simulink model "testemplanner_cs"  (R2020a)
settings: Solver=ode5  StartTime=0.0  StopTime=24  FixedStep=1/1000  RelTol=1e-3
PreLoadFcn:
  | mbxruntime.callbacks.PreLoadFcn(bdroot);
PostLoadFcn:
  | mbxruntime.callbacks.PostLoadFcn(bdroot);
InitFcn:
  | mbxruntime.callbacks.InitFcn(bdroot);
StartFcn:
  | mbxruntime.callbacks.StartFcn(bdroot);
StopFcn:
  | mbxruntime.callbacks.StopFcn(bdroot);
model workspace (MAT data in the model file):
  mbox_table : object (value not decoded)
  model_closed = 0
  sim_status = 0
values from neighbouring files (symbols this model uses):
  c_factor = 43.75    [emplanner_init.m]
  cf = -175016    [emplanner_init.m]
  cr = -130634    [emplanner_init.m]
  global_path_x = [0.057304 1.05668625507 2.05480936558 3.05165624935 4.04722112279 5.04150235808 6.03449985569 7.02621407764 8.01664569183 9.00579544113 9.99366409523 10.9802524329 ... (3001 elements, 3001x1)]    [global_path.mat]
  global_path_y = [8.29 8.29 8.29 8.29 8.29 8.29 8.29 8.29 8.29 8.29 8.29 8.29 ... (3001 elements, 3001x1)]    [global_path.mat]
  KD_PID_distance = 0.0    (= 0)    [emplanner_init.m]
  KD_PID_speed = 0    [emplanner_init.m]
  KI_PID_distance = 0.0    (= 0)    [emplanner_init.m]
  KI_PID_speed = 0    [emplanner_init.m]
  KP_PID_distance = 0.5    [emplanner_init.m]
  KP_PID_speed = 1.8    [emplanner_init.m]
  la = 1.265    [emplanner_init.m]
  lb = 2.947-1.265    (= 1.682)    [emplanner_init.m]
  LQR_K1 = k(:,1)'    [emplanner_init.m]
  LQR_K2 = k(:,2)'    [emplanner_init.m]
  LQR_K3 = k(:,3)'    [emplanner_init.m]
  LQR_K4 = k(:,4)'    [emplanner_init.m]
  m = 2020    [emplanner_init.m]
  rack_displacement = [-39.14 , -37.2 , -35.29 , -33.43 , -31.6 , -29.81 , -28.06 , -26.34 , -24.66 ,      -23.01 , -21.38 , -19.79 , -18.23 , -16.69 , -15.18 , -13.7 , -12.23 , -10.8 , -9.38 , -7.98 ,     -6.61 , -5.25 , -3.91 , -2.59 , -1.29 , 0 , 1.27 , 2.54 , 3.78 , 5.02 , 6.24 , 7.46 , 8.66 ,      9.86 , 11.05 , 12.24 , 13.41 , 14.59 , 15.76 , 16.92 , 18.09 , 19.25 , 20.42 , 21.59 , 22.76 ,      23.93 , 25.11 , 26 ...(+26 chars)    [emplanner_init.m]
  right_wheel_ground = [-70 ,-67.2 , -64.4 , -61.6 , -58.8 , -56 , -53.2 , -50.4 , -47.6 , -44.8 , -42 ,      -39.2 , -36.4 , -33.6 , -30.8 , -28 , -25.2 , -22.4 , -19.6 , -16.8 , -14 , -11.2 , -8.4 , -5.6 ,      -2.8 , 0 , 2.8 , 5.6 , 8.4 , 11.2 , 14 , 16.8 , 19.6 , 22.4 , 25.2 , 28 , 30.8 , 33.6 , 36.4 ,      39.2 , 42 , 44.8 , 47.6 , 50.4 , 53.2 , 56 , 58.8 , 61.6 , 64.4 , 67.2 , 70 ]    [emplanner_init.m]
  vx_break_point = zeros(1,5000)    [emplanner_init.m]
undefined symbols (not defined in the file or in its folder): aubr, DiscIntNeverNeededParam, tablebr, vubr
libraries: PreScanSimulinkLibrary x9, Solver_SF x1, simulink_extras x1
(part 9 of 9)

== matlab function testemplanner_cs/Audi_A8_Sedan_1/decision&planning module/EM_planner1/DP path1 ==
  data: plan_start_s input; dp_path_s_init output; plan_start_l input; plan_start_dl input; plan_start_ddl input; obs_s_set input; obs_l_set input; w_smooth_dl_cost input; w_collision_cost input; w_ref_cost input; w_smooth_ddl_cost input; w_smooth_dddl_cost input; col input; row input; sample_s input; sample_l input; dp_path_l_init output
function [dp_path_s_init,dp_path_l_init] = fcn(plan_start_s,plan_start_l,plan_start_dl,plan_start_ddl,obs_s_set,obs_l_set,w_smooth_dl_cost,w_collision_cost,w_ref_cost,w_smooth_ddl_cost,w_smooth_dddl_cost,col,row,sample_s,sample_l)
%%作用：撒点，通过动态规划算出代价最小的路径点集合，算出要进行优化的凸空间
%%输入：规划起点的s，l,dl,ddl,静态障碍物的s，l集合，dl，ddl，dddl平滑代价，参考线代价以及碰撞代价权重
%%行数：为奇数，列数；采样的横向距离以及纵向距离

%%输出：计算得到的路径点s，l初始值

%首先定义一个代价数组，代表从起点到当前i，j点的总代价，均初始化为inf无穷大
node=ones(row,col)*inf;

%再定义一个pre_node,用来表征node的父节点的坐标索引，均初始化为0，0；假设所有节点的父节点均为起点

pre_node=zeros(row,col);
%首先计算第一列的点的cost，调用CalccostFromStart函数进行计算
for i=1:row
    node(i,1)=CalccostFromStart(plan_start_s,plan_start_l,plan_start_dl,plan_start_ddl,obs_s_set,obs_l_set,w_smooth_dl_cost,w_collision_cost,w_ref_cost,w_smooth_ddl_cost,w_smooth_dddl_cost,i,row,sample_s,sample_l);
end
%计算从第二列开始的每一列的最小代价值以及其父节点的索引值，调用CalccostFromNeibor函数进行计算
for j=2:col
    for k =1:row
    [node,pre_node]=CalccostFromNeibor(plan_start_s,node,pre_node,k,j,obs_s_set,obs_l_set,w_smooth_dl_cost,w_collision_cost,w_ref_cost,w_smooth_ddl_cost,w_smooth_dddl_cost,row,sample_s,sample_l);
    end
end
% 找到最后一列中代价最小的节点
min_cost=node(1,end);
index=1;
for i=2:row
    min_cost_temp=node(i,end);
    if min_cost_temp<min_cost
        index=i;
        min_cost=min_cost_temp;
    else
    end
end

%因为不知道有多少个点，所以做一个缓冲
dp_path_s_init=ones(15,1)* -1;
dp_path_l_init=ones(15,1)* -1;

temp_node=zeros(15,1);

%从最后一个节点开始，反向找到最小代价路径上的所有点，并放入集合中
for i=col:-1:1
    
    temp_node(i)=pre_node(index,i);
    index=pre_node(index,i);
end
%确定路径上点的s，l值
for i=1:col
dp_path_s_init(i)=sample_s*i;
dp_path_l_init(i)=sample_l*(temp_node(col+1-i)-(row+1)/2);
end
end

%函数CalccostFromNeibor，计算从上一列的临近点到这个点的最小cost值和其父节点的行索引
function [node,pre_node]=CalccostFromNeibor(plan_start_s,node,pre_node,k,j,obs_s_set,obs_l_set,w_smooth_dl_cost,w_collision_cost,w_ref_cost,w_smooth_ddl_cost,w_smooth_dddl_cost,row,sample_s,sample_l)
% %作用： 计算从从上一列的临近点到这个点的最小cost值和其父节点的行索引
  %输入：起点的s，l，障碍物的s,l,dl,ddl,dddl平滑权重，障碍物碰撞权重，参考线权重，当前所在行数，列数，总行数，采样s，l，node和pre_node数组
  %输出：更新后的node和pre_node数组
  %dl，ddl设为0，因为DP仅仅是为了粗略开辟凸空间，不用太精细。
start_s=plan_start_s+sample_s*(j-1);
end_s=start_s+plan_start_s+sample_s*(j);
start_dl=0;
start_ddl=0;
end_dl=0;
end_ddl=0;
cost=zeros(row,1);
%确定起点和终点参数，计算五次多项式系数
for i=1:row
start_l=sample_l*(i-(row+1)/2);
end_l=sample_l*(k-(row+1)/2);
%调用函数计算五次多项式系数
coffee=Calccoffee(start_s,start_l,start_dl,start_ddl,end_s,end_l,end_dl,end_ddl);

s_set=zeros(10,1);
l_set=zeros(10,1);
dl_set=zeros(10,1);
ddl_set=zeros(10,1);
dddl_set=zeros(10,1);

%找10个点进行代价计算
for n=1:10
    s_set(n)=start_s+sample_s/10*(n-1);
    l_set(n)=coffee(1)*(s_set(n))^5+coffee(2)*(s_set(n))^4+coffee(3)*(s_set(n))^3+coffee(4)*(s_set(n))^2+coffee(5)*(s_set(n))+coffee(6);
    dl_set(n)=5*coffee(1)*(s_set(n))^4+4*coffee(2)*(s_set(n))^3+3*coffee(3)*(s_set(n))^2+2*coffee(4)*(s_set(n))+coffee(5);
    ddl_set(n)=20*coffee(1)*(s_set(n))^3+12*coffee(2)*(s_set(n))^2+6*coffee(3)*(s_set(n))+2*coffee(4);
    dddl_set(n)=60*coffee(1)*(s_set(n))^2+24*coffee(2)*(s_set(n))+6*coffee(3);
end
%首先计算平滑带代价和参考线代价
smooth_cost=w_smooth_dl_cost*(dl_set'*dl_set)+w_smooth_ddl_cost*(ddl_set'*ddl_set)+w_smooth_dddl_cost*(dddl_set'*dddl_set);
ref_cost=w_ref_cost*(l_set'*l_set);
%接着计算障碍物代价
collision_cost=0;
for m=1:length(obs_s_set)
    if isnan(obs_s_set(m))
        break;
    end
    s_err=obs_s_set(m)*ones(10,1)-s_set;
    l_err=obs_l_set(m)*ones(10,1)-l_set;
    err_squard=s_err.^2+l_err.^2;
    %调用障碍物代价模型函数CalcObsCost进行计算
    collision_cost_one=CalcObsCost(err_squard,w_collision_cost);
    collision_cost=collision_cost+collision_cost_one;
end

cost(i)=smooth_cost+ref_cost+collision_cost+node(i,j-1);
end
index=1;
min_cost=cost(1);
for h =2:row
   
    min_cost_temp=cost(h);
    if min_cost_temp<min_cost
        index=h;
        min_cost=min_cost_temp;
    else
    end
end
 pre_node(k,j)=index;
 node(k,j)=min_cost;
end




%函数CalccostFromStart，计算从起点到第一列的点的cost值
function cost=CalccostFromStart(plan_start_s,plan_start_l,plan_start_dl,plan_start_ddl,obs_s_set,obs_l_set,w_smooth_dl_cost,w_collision_cost,w_ref_cost,w_smooth_ddl_cost,w_smooth_dddl_cost,node_row,row,sample_s,sample_l)

  %作用： 计算从起点到第一列的点的cost值
  %输入：起点的s，l，dl，ddl,障碍物的s,l,dl,ddl,dddl平滑权重，障碍物碰撞权重，参考线权重，当前所在行数，总行数，采样s，l
  %输出：代价和
start_s=plan_start_s;
start_l=plan_start_l;
start_dl=plan_start_dl;
start_ddl=plan_start_ddl;
end_s=start_s+sample_s;
end_l=sample_l*(node_row-(row+1)/2);
end_dl=0;
end_ddl=0;
%调用函数计算五次多项式系数
coffee=Calccoffee(start_s,start_l,start_dl,start_ddl,end_s,end_l,end_dl,end_ddl);

s_set=zeros(10,1);
l_set=zeros(10,1);
dl_set=zeros(10,1);
ddl_set=zeros(10,1);
dddl_set=zeros(10,1);

%找10个点进行代价计算
for i=1:10
    s_set(i)=start_s+sample_s/10*(i-1);
    l_set(i)=coffee(1)*(s_set(i))^5+coffee(2)*(s_set(i))^4+coffee(3)*(s_set(i))^3+coffee(4)*(s_set(i))^2+coffee(5)*(s_set(i))+coffee(6);
    dl_set(i)=5*coffee(1)*(s_set(i))^4+4*coffee(2)*(s_set(i))^3+3*coffee(3)*(s_set(i))^2+2*coffee(4)*(s_set(i))+coffee(5);
    ddl_set(i)=20*coffee(1)*(s_set(i))^3+12*coffee(2)*(s_set(i))^2+6*coffee(3)*(s_set(i))+2*coffee(4);
    dddl_set(i)=60*coffee(1)*(s_set(i))^2+24*coffee(2)*(s_set(i))+6*coffee(3);
end
%首先计算平滑带代价和参考线代价
smooth_cost=w_smooth_dl_cost*(dl_set'*dl_set)+w_smooth_ddl_cost*(ddl_set'*ddl_set)+w_smooth_dddl_cost*(dddl_set'*dddl_set);
ref_cost=w_ref_cost*(l_set'*l_set);
%接着计算障碍物代价
collision_cost=0;
for i=1:length(obs_s_set)
    if isnan(obs_s_set(i))
        break;
    end
    s_err=obs_s_set(i)*ones(10,1)-s_set;
    l_err=obs_l_set(i)*ones(10,1)-l_set;
    err_squard=s_err.^2+l_err.^2;
     %调用障碍物代价模型函数CalcObsCost进行计算
    collision_cost_one=CalcObsCost(err_squard,w_collision_cost);
    collision_cost=collision_cost+collision_cost_one;
end

cost=smooth_cost+ref_cost+collision_cost;


end
function coffee=Calccoffee(start_s,start_l,start_dl,start_ddl,end_s,end_l,end_dl,end_ddl)
  %作用：计算五次多项式系数
  %输入：起点和终点的s,l,dl,ddl共6个值
  %输出：六个权重系数
    start_s2=start_s*start_s;
    start_s3=start_s2*start_s;
    start_s4=start_s3*start_s;
    start_s5=start_s4*start_s;
    end_s2=end_s*end_s;
    end_s3=end_s2*end_s;
    end_s4=end_s3*end_s;
    end_s5=end_s4*end_s;
    A=[1,start_s,start_s2,start_s3,start_s4,start_s5;
       0,1,2*start_s,3*start_s2,4*start_s3,5*start_s4;
       0,0,2,6*start_s,12*start_s2,20*start_s3;
       1,end_s,end_s2,end_s3,end_s4,end_s5;
       0,1,2*end_s,3*end_s2,4*end_s3,5*end_s4;
        0,0,2,6*end_s,12*end_s2,20*end_s3;];
    B=[start_l;start_dl;start_ddl;end_l;end_dl;end_ddl];
    coffee=A\B;
end
function obscost=CalcObsCost(err_squard,w_collision_cost)
  %作用： %建立一个障碍物评估模型，进行代价评估
  %输入：与障碍物的横纵向距离平方和，碰撞权重
  %输出：障碍物代价和
    cost=0;
    for i=1:length(err_squard)
        if err_squard(i)>16
        elseif err_squard(i)<=16 &&err_squard(i)>=9
            cost=cost+1000/err_squard(i);
        else
            cost=cost+w_collision_cost;
        end
    end
    obscost=cost;
end

== matlab function testemplanner_cs/Audi_A8_Sedan_1/decision&planning module/EM Planner/Cartesian2Frenet1/MATLAB Function1 ==
  data: l_set input; s_dot_set output; vx_set input; vy_set input; proj_heading_set input; proj_kappa_set input; l_dot_set output; dl_set output
function [s_dot_set,l_dot_set,dl_set] = fcn(l_set,vx_set,vy_set,proj_heading_set,proj_kappa_set)
%该函数将计算frenet坐标系下的s_dot, l_dot, dl/ds
n = 128;
% 输出初始化
s_dot_set = ones(n,1)*nan;
l_dot_set = ones(n,1)*nan;
dl_set = ones(n,1)*nan;

for i = 1 : length(l_set)
    if isnan(l_set(i))
        break;
    end
    v_h = [vx_set(i);vy_set(i)];
    n_r = [-sin(proj_heading_set(i));cos(proj_heading_set(i))];
    t_r = [cos(proj_heading_set(i));sin(proj_heading_set(i))];
    l_dot_set(i) = v_h'*n_r;
    s_dot_set(i) = v_h'*t_r/(1 - proj_kappa_set(i)*l_set(i));
    %%%向量法做cartesian与frenet的转换要更简单，但是也有缺点，向量法必须依赖速度加速度
    %l' = l_dot/s_dot 但是如果s_dot = 0 此方法就失效了
    if abs(s_dot_set(i)) < 1e-6
        dl_set(i) = 0;
    else
        dl_set(i) = l_dot_set(i)/s_dot_set(i);
    end
end

== matlab function testemplanner_cs/Audi_A8_Sedan_1/decision&planning module/EM_planner1/Frenet2Cart ==
  data: s_set input; x_set output; l_set input; dl_set input; ddl_set input; frenet_s input; frenet_l input; frenet_heading input; frenet_kappa input; index2s input; y_set output; heading_set output; kappa_set output
function [x_set,y_set,heading_set,kappa_set] = fcn(s_set,l_set,dl_set,ddl_set,frenet_s,frenet_l,frenet_heading,frenet_kappa,index2s)

%%作用：实现frenet坐标转换为笛卡尔坐标，进行控制.整个流程是先根据s求匹配点的x,y，再根据ds求投影点的x，y,再根据dl求要转换点的x,y
%%输入：frenet坐标下路径的s，l,dl,ddl;参考线的s,l,heading,kappa以及index2s

%%输出：路径在笛卡尔坐标系下的x,y,heading,kappa

%不知道要转换多少个点，因此进行缓冲

n=128;
%初始化输出
x_set=ones(n,1)*nan;
y_set=ones(n,1)*nan;
heading_set=ones(n,1)*nan;
kappa_set=ones(n,1)*nan;
for i=1:length(s_set)
    if isnan(s_set(i))
        break;
    end
    %写一个函数，用来计算路径s,l所对应的投影点的直角坐标系x，y，heading，kappa
    [proj_x,proj_y,proj_heading,proj_kappa]=calcProjPoint(s_set(i),frenet_s,frenet_l,frenet_heading,frenet_kappa,index2s);
    nor=[-sin(proj_heading);cos(proj_heading)];
    point_cert=[proj_x;proj_y]+l_set(i)*nor;
    x_set(i)=point_cert(1);
    y_set(i)=point_cert(2);
    heading_set(i) = proj_heading + atan(dl_set(i)/(1 - proj_kappa * l_set(i)));
    % 近似认为 kappa' == 0,frenet转cartesian公式，见第一章第三节评论区的链接
    kappa_set(i) = ((ddl_set(i) + proj_kappa * dl_set(i) * tan(heading_set(i) - proj_heading)) * ...
        (cos(heading_set(i) - proj_heading)^2)/(1 - proj_kappa * l_set(i)) + proj_kappa) * ...
        cos(heading_set(i) - proj_heading)/(1 - proj_kappa * l_set(i));
    
end
end


function  [proj_x,proj_y,proj_heading,proj_kappa]=calcProjPoint(s,frenet_x,frenet_y,frenet_heading,frenet_kappa,index2s)
   
    match_point_index = 1;
    while index2s(match_point_index) < s
        match_point_index = match_point_index + 1;
    end
    ds=s-index2s(match_point_index);
    tor=[cos(frenet_heading(match_point_index));sin(frenet_heading(match_point_index))];
    point=[frenet_x((match_point_index));frenet_y((match_point_index))]+ds*tor;
    proj_x=point(1);
    proj_y=point(2);
    proj_heading=frenet_heading((match_point_index))+ds*frenet_kappa(match_point_index);
    proj_kappa=frenet_kappa(match_point_index);
    end

== matlab function testemplanner_cs/Audi_A8_Sedan_1/decision&planning module/EM_planner1/Index to s ==
  data: path_x input; index2s output; path_y input; origin_point_x input; origin_point_y input; origin_match_point_index input
function index2s = fcn(path_x,path_y,origin_point_x,origin_point_y,origin_match_point_index)
    
%作用：求出frenet坐标系下的点在世界坐标系下通过index所对应的s值，即index2s
%输入：参考线、frenet坐标原点的坐标，frenet坐标原点所对应的匹配点的index
%输出：index2s：index和s之间的对应关系

%首先定义index2s数组
n=181;
index2s=zeros(181,1);

%首先计算以path起点为原点的index2s值
for i=2:n
    index2s(i)=sqrt((path_x(i)-path_x(i-1))^2+(path_y(i)-path_y(i-1))^2)+index2s(i-1);
end

%再计算从path起点到匹配点的距离S0，用上面计算的index2s减去S0即可得出真实的index2s
%s_temp =  index2s(origin_match_point_index);
%调用函数，计算路径起点的index所对应的弧长s
s = CalcSfromIndex(path_x,path_y,origin_point_x,origin_point_y,origin_match_point_index,index2s);  
%用当前点到坐标原点的s减去路径起点到坐标原点的S，就是最终的距离路径起点的s
index2s=index2s-s*ones(n,1);
end
 function s=CalcSfromIndex(ref_path_x,ref_path_y,match_point_x,match_point_y,match_point_index,index2s)   %使用一个函数来计算index所对应的S值
%%首先判断原点是在匹配点前还是匹配点后，通过向量的内积来进行判断
s_temp =  index2s(match_point_index);
vector1=[match_point_x-ref_path_x(match_point_index);match_point_y-ref_path_y(match_point_index)];
%考虑匹配点在路径终点的情况，不在终点就是匹配点和下一个点作为方向向量，如果是终点则使用匹配点和上一个点作为方向向量
if match_point_index<length(ref_path_x)
    vector2=[ref_path_x(match_point_index+1)-ref_path_x(match_point_index);ref_path_y(match_point_index+1)-ref_path_y(match_point_index)];
else
     vector2=[ref_path_x(match_point_index)-ref_path_x(match_point_index-1);ref_path_y(match_point_index)-ref_path_y(match_point_index-1)];
end
result=vector1'*vector2;    
if result >0 %原点在匹配点后，加上这个距离
    s=s_temp+sqrt(vector1'*vector1);
else        %原点在匹配点前，减去这个距离
    s=s_temp-sqrt(vector1'*vector1);
end
end

== matlab function testemplanner_cs/Audi_A8_Sedan_1/decision&planning module/EM_planner1/MATLAB Function ==
  data: s input; l input
function fcn(s,l)
coder.extrinsic("plot")
plot(s,l);

== matlab function testemplanner_cs/Audi_A8_Sedan_1/decision&planning module/EM_planner1/MATLAB Function1 ==
  data: x_set input; match_point_index_set output; y_set input; frenet_path_x input; frenet_path_y input; frenet_path_heading input; frenet_path_kappa input; proj_x_set output; proj_y_set output; proj_heading_set output; proj_kappa_set output
function [match_point_index_set,proj_x_set, proj_y_set,proj_heading_set,proj_kappa_set] = ...
    fcn(x_set,y_set,frenet_path_x,frenet_path_y,frenet_path_heading,frenet_path_kappa)
%该函数将批量计算x_set，y_set中的xy，在frenet_path下的投影的信息
%输入 x_set,y_set，待投影的点的集合
%x_set,y_set,frenet_path_x,frenet_path_y,frenet_path_heading,frenet_path_kappa
%曲线在直角坐标系下的x，y，heading，kappa
%输出：match_point_index_set 匹配点在frenet_path下的编号的集合(即从全局路径第一个点开始数，第几个点是匹配点)
%     proj_x y heading kappa 投影的x,y,heading,kappa的集合

% 由于事先不知道x_set中到底有多少个点需要投影，因此事先声明一个最大的数量的点作为缓冲
n = 128;
% 并且由于不知道投影点的个数，所以也不知道输出的个数，因此输出也要做缓冲，用nan表示不存在的点
% 输出最多输出128个
% 输出初始化
match_point_index_set = ones(n,1) * nan;
proj_x_set = ones(n,1) * nan;
proj_y_set = ones(n,1) * nan;
proj_heading_set = ones(n,1) * nan;
proj_kappa_set = ones(n,1) * nan;

%找匹配点，需要利用上一个周期的结果作为下一个周期遍历的起点，因此需要声明两个全局变量
persistent is_first_run;
persistent pre_match_point_index_set;
persistent pre_frenet_path_x;
persistent pre_frenet_path_y;
persistent pre_frenet_path_heading;
persistent pre_frenet_path_kappa;
%算法主函数入口

if isempty(is_first_run)
    %该if分支表示函数首次运行
    is_first_run = 0;
    pre_frenet_path_x = frenet_path_x;
    pre_frenet_path_y = frenet_path_y;
    pre_frenet_path_heading = frenet_path_heading;
    pre_frenet_path_kappa = frenet_path_kappa;
    %要记录首次运行计算的匹配点的结果供下个周期运行，先初始化
    pre_match_point_index_set = ones(n,1) * nan;
    %对x_set,y_set的点做遍历，找到他们的匹配点
    for i = 1 : length(x_set)
        if isnan(x_set(i))
            break;
        end
        %首次运行时，没有任何提示，只能从frenet path的第一个点开始找
        start_search_index = 1;
        % 声明increase_count，用于表示在遍历时distance连续增加的个数
        increase_count = 0;
        % 开始遍历
        min_distance = inf;
        for j = start_search_index : length(frenet_path_x)
            distance = (x_set(i) - frenet_path_x(j))^2 + (y_set(i) - frenet_path_y(j))^2;
            if distance < min_distance
                min_distance = distance;
                match_point_index_set(i) = j;
                increase_count = 0;
            else
                increase_count = increase_count + 1;
            end
            %如果distance连续增加50次就不要再遍历了，节省时间
            if increase_count > 50
                break;
            end
        end
        
        %如何通过匹配点计算投影点，请参见《自动驾驶控制算法第七讲》
        %或《自动驾驶决策规划算法》第一章第三节
        
        %取出匹配点的编号
        match_point_index = match_point_index_set(i);
        %取出匹配点的信息
        match_point_x = frenet_path_x(match_point_index);
        match_point_y = frenet_path_y(match_point_index);
        match_point_heading = frenet_path_heading(match_point_index);
        match_point_kappa = frenet_path_kappa(match_point_index);
        %计算匹配点的方向向量与法向量
        vector_match_point = [match_point_x;match_point_y];
        vector_match_point_direction = [cos(match_point_heading);sin(match_point_heading)];
        %声明待投影点的位矢
        vector_r = [x_set(i);y_set(i)];
        
       %通过匹配点计算投影点
       vector_d = vector_r - vector_match_point;
       ds = vector_d' * vector_match_point_direction;
       vector_proj_point = vector_match_point + ds * vector_match_point_direction;
       proj_heading = match_point_heading + match_point_kappa * ds;
       proj_kappa = match_point_kappa;
       %计算结果输出
       proj_x_set(i) = vector_proj_point(1);
       proj_y_set(i) = vector_proj_point(2);
       proj_heading_set(i) = proj_heading;
       proj_kappa_set(i) = proj_kappa;
    end
    %匹配点的计算结果保存，供下一个周期使用
    pre_match_point_index_set = match_point_index_set;
else
    %此if分支表示不是首次运行
    
    %对每个x_set上的点做处理
    for i = 1 : length(x_set)
        %不是首次运行，对于点x_set(i),y_set(i)来说,start_search_index =
        %pre_match_point_index_set(i)
        start_search_index = pre_match_point_index_set(i);%上个周期匹配点的编号作为本周期搜索的起点
        % 声明increase_count，用于表示在遍历时distance连续增加的个数
        %%%%%%%%%
        %对于障碍物检测而言，当感知第一次检测到障碍物时，算法并不是首次运行，此时 
        %pre_match_point_index_set的值是nan，如果还用上一时刻的结果作为本周期搜索的起点
        %必然会出问题，所以要修改
        % 声明increase_count_limit
        increase_count_limit = 5;
        if isnan(start_search_index)
            %没有上个周期的结果，那就不能只检查5次了
            increase_count_limit = 50;
            %搜索起点也要设为1
            start_search_index = 1;
        end
        increase_count = 0;
        % 开始遍历
        %这里多一个步骤，判断遍历的方向
        %计算上个周期匹配点的位矢
        vector_pre_match_point = [pre_frenet_path_x(start_search_index);pre_frenet_path_y(start_search_index)];
        vector_pre_match_point_direction = ...
            [cos(pre_frenet_path_heading(start_search_index));sin(pre_frenet_path_heading(start_search_index))];
        %判断遍历的方向
        flag = ([x_set(i);y_set(i)] - vector_pre_match_point)' * vector_pre_match_point_direction;
        min_distance = inf;
        if flag > 0.001
            for j = start_search_index : length(frenet_path_x)
                distance = (x_set(i) - frenet_path_x(j))^2 + (y_set(i) - frenet_path_y(j))^2;
                if distance < min_distance
                    min_distance = distance;
                    match_point_index_set(i) = j;
                    increase_count = 0;
                else
                    increase_count = increase_count + 1;
                end
                %如果distance连续增加increase_count_limit次就不要再遍历了，节省时间
                if increase_count > increase_count_limit
                    break;
                end
            end
        elseif flag < - 0.001
            for j = start_search_index : -1 : 1
                distance = (x_set(i) - frenet_path_x(j))^2 + (y_set(i) - frenet_path_y(j))^2;
                if distance < min_distance
                    min_distance = distance;
                    match_point_index_set(i) = j;
                    increase_count = 0;
                else
                    increase_count = increase_count + 1;
                end
                %如果distance连续增加increase_count_limit次就不要再遍历了，节省时间
                if increase_count > increase_count_limit
                    break;
                end
            end
        else
            match_point_index_set(i) = start_search_index;
        end
        
        %如何通过匹配点计算投影点，请参见《自动驾驶控制算法第七讲》
        %或《自动驾驶决策规划算法》第一章第三节
        
        %取出匹配点的编号
        match_point_index = match_point_index_set(i);
        %取出匹配点的信息
        match_point_x = frenet_path_x(match_point_index);
        match_point_y = frenet_path_y(match_point_index);
        match_point_heading = frenet_path_heading(match_point_index);
        match_point_kappa = frenet_path_kappa(match_point_index);
        %计算匹配点的方向向量与法向量
        vector_match_point = [match_point_x;match_point_y];
        vector_match_point_direction = [cos(match_point_heading);sin(match_point_heading)];
        %声明待投影点的位矢
        vector_r = [x_set(i);y_set(i)];
        
       %通过匹配点计算投影点
       vector_d = vector_r - vector_match_point;
       ds = vector_d' * vector_match_point_direction;
       vector_proj_point = vector_match_point + ds * vector_match_point_direction;
       proj_heading = match_point_heading + match_point_kappa * ds;
       proj_kappa = match_point_kappa;
       %计算结果输出
       proj_x_set(i) = vector_proj_point(1);
       proj_y_set(i) = vector_proj_point(2);
       proj_heading_set(i) = proj_heading;
       proj_kappa_set(i) = proj_kappa;
  
    end
    %匹配点的计算结果保存，供下一个周期使用
    pre_match_point_index_set = match_point_index_set;
    pre_frenet_path_x = frenet_path_x;
    pre_frenet_path_y = frenet_path_y;
    pre_frenet_path_heading = frenet_path_heading;
    pre_frenet_path_kappa = frenet_path_kappa;
end

== matlab function testemplanner_cs/Audi_A8_Sedan_1/decision&planning module/EM_planner1/MATLAB Function2 ==
  data: x_set input; match_point_index_set output; y_set input; frenet_path_x input; frenet_path_y input; frenet_path_heading input; frenet_path_kappa input; proj_x_set output; proj_y_set output; proj_heading_set output; proj_kappa_set output
function [match_point_index_set,proj_x_set, proj_y_set,proj_heading_set,proj_kappa_set] = ...
    fcn(x_set,y_set,frenet_path_x,frenet_path_y,frenet_path_heading,frenet_path_kappa)
%该函数将批量计算x_set，y_set中的xy，在frenet_path下的投影的信息
%输入 x_set,y_set，待投影的点的集合
%x_set,y_set,frenet_path_x,frenet_path_y,frenet_path_heading,frenet_path_kappa
%曲线在直角坐标系下的x，y，heading，kappa
%输出：match_point_index_set 匹配点在frenet_path下的编号的集合(即从全局路径第一个点开始数，第几个点是匹配点)
%     proj_x y heading kappa 投影的x,y,heading,kappa的集合

% 由于事先不知道x_set中到底有多少个点需要投影，因此事先声明一个最大的数量的点作为缓冲
n = 128;
% 并且由于不知道投影点的个数，所以也不知道输出的个数，因此输出也要做缓冲，用nan表示不存在的点
% 输出最多输出128个
% 输出初始化
match_point_index_set = ones(n,1) * nan;
proj_x_set = ones(n,1) * nan;
proj_y_set = ones(n,1) * nan;
proj_heading_set = ones(n,1) * nan;
proj_kappa_set = ones(n,1) * nan;

%找匹配点，需要利用上一个周期的结果作为下一个周期遍历的起点，因此需要声明两个全局变量
persistent is_first_run;
persistent pre_match_point_index_set;
persistent pre_frenet_path_x;
persistent pre_frenet_path_y;
persistent pre_frenet_path_heading;
persistent pre_frenet_path_kappa;
%算法主函数入口

if isempty(is_first_run)
    %该if分支表示函数首次运行
    is_first_run = 0;
    pre_frenet_path_x = frenet_path_x;
    pre_frenet_path_y = frenet_path_y;
    pre_frenet_path_heading = frenet_path_heading;
    pre_frenet_path_kappa = frenet_path_kappa;
    %要记录首次运行计算的匹配点的结果供下个周期运行，先初始化
    pre_match_point_index_set = ones(n,1) * nan;
    %对x_set,y_set的点做遍历，找到他们的匹配点
    for i = 1 : length(x_set)
        if isnan(x_set(i))
            break;
        end
        %首次运行时，没有任何提示，只能从frenet path的第一个点开始找
        start_search_index = 1;
        % 声明increase_count，用于表示在遍历时distance连续增加的个数
        increase_count = 0;
        % 开始遍历
        min_distance = inf;
        for j = start_search_index : length(frenet_path_x)
            distance = (x_set(i) - frenet_path_x(j))^2 + (y_set(i) - frenet_path_y(j))^2;
            if distance < min_distance
                min_distance = distance;
                match_point_index_set(i) = j;
                increase_count = 0;
            else
                increase_count = increase_count + 1;
            end
            %如果distance连续增加50次就不要再遍历了，节省时间
            if increase_count > 50
                break;
            end
        end
        
        %如何通过匹配点计算投影点，请参见《自动驾驶控制算法第七讲》
        %或《自动驾驶决策规划算法》第一章第三节
        
        %取出匹配点的编号
        match_point_index = match_point_index_set(i);
        %取出匹配点的信息
        match_point_x = frenet_path_x(match_point_index);
        match_point_y = frenet_path_y(match_point_index);
        match_point_heading = frenet_path_heading(match_point_index);
        match_point_kappa = frenet_path_kappa(match_point_index);
        %计算匹配点的方向向量与法向量
        vector_match_point = [match_point_x;match_point_y];
        vector_match_point_direction = [cos(match_point_heading);sin(match_point_heading)];
        %声明待投影点的位矢
        vector_r = [x_set(i);y_set(i)];
        
       %通过匹配点计算投影点
       vector_d = vector_r - vector_match_point;
       ds = vector_d' * vector_match_point_direction;
       vector_proj_point = vector_match_point + ds * vector_match_point_direction;
       proj_heading = match_point_heading + match_point_kappa * ds;
       proj_kappa = match_point_kappa;
       %计算结果输出
       proj_x_set(i) = vector_proj_point(1);
       proj_y_set(i) = vector_proj_point(2);
       proj_heading_set(i) = proj_heading;
       proj_kappa_set(i) = proj_kappa;
    end
    %匹配点的计算结果保存，供下一个周期使用
    pre_match_point_index_set = match_point_index_set;
else
    %此if分支表示不是首次运行
    
    %对每个x_set上的点做处理
    for i = 1 : length(x_set)
        %不是首次运行，对于点x_set(i),y_set(i)来说,start_search_index =
        %pre_match_point_index_set(i)
        start_search_index = pre_match_point_index_set(i);%上个周期匹配点的编号作为本周期搜索的起点
        % 声明increase_count，用于表示在遍历时distance连续增加的个数
        %%%%%%%%%
        %对于障碍物检测而言，当感知第一次检测到障碍物时，算法并不是首次运行，此时 
        %pre_match_point_index_set的值是nan，如果还用上一时刻的结果作为本周期搜索的起点
        %必然会出问题，所以要修改
        % 声明increase_count_limit
        increase_count_limit = 5;
        if isnan(start_search_index)
            %没有上个周期的结果，那就不能只检查5次了
            increase_count_limit = 50;
            %搜索起点也要设为1
            start_search_index = 1;
        end
        increase_count = 0;
        % 开始遍历
        %这里多一个步骤，判断遍历的方向
        %计算上个周期匹配点的位矢
        vector_pre_match_point = [pre_frenet_path_x(start_search_index);pre_frenet_path_y(start_search_index)];
        vector_pre_match_point_direction = ...
            [cos(pre_frenet_path_heading(start_search_index));sin(pre_frenet_path_heading(start_search_index))];
        %判断遍历的方向
        flag = ([x_set(i);y_set(i)] - vector_pre_match_point)' * vector_pre_match_point_direction;
        min_distance = inf;
        if flag > 0.001
            for j = start_search_index : length(frenet_path_x)
                distance = (x_set(i) - frenet_path_x(j))^2 + (y_set(i) - frenet_path_y(j))^2;
                if distance < min_distance
                    min_distance = distance;
                    match_point_index_set(i) = j;
                    increase_count = 0;
                else
                    increase_count = increase_count + 1;
                end
                %如果distance连续增加increase_count_limit次就不要再遍历了，节省时间
                if increase_count > increase_count_limit
                    break;
                end
            end
        elseif flag < - 0.001
            for j = start_search_index : -1 : 1
                distance = (x_set(i) - frenet_path_x(j))^2 + (y_set(i) - frenet_path_y(j))^2;
                if distance < min_distance
                    min_distance = distance;
                    match_point_index_set(i) = j;
                    increase_count = 0;
                else
                    increase_count = increase_count + 1;
                end
                %如果distance连续增加increase_count_limit次就不要再遍历了，节省时间
                if increase_count > increase_count_limit
                    break;
                end
            end
        else
            match_point_index_set(i) = start_search_index;
        end
        
        %如何通过匹配点计算投影点，请参见《自动驾驶控制算法第七讲》
        %或《自动驾驶决策规划算法》第一章第三节
        
        %取出匹配点的编号
        match_point_index = match_point_index_set(i);
        %取出匹配点的信息
        match_point_x = frenet_path_x(match_point_index);
        match_point_y = frenet_path_y(match_point_index);
        match_point_heading = frenet_path_heading(match_point_index);
        match_point_kappa = frenet_path_kappa(match_point_index);
        %计算匹配点的方向向量与法向量
        vector_match_point = [match_point_x;match_point_y];
        vector_match_point_direction = [cos(match_point_heading);sin(match_point_heading)];
        %声明待投影点的位矢
        vector_r = [x_set(i);y_set(i)];
        
       %通过匹配点计算投影点
       vector_d = vector_r - vector_match_point;
       ds = vector_d' * vector_match_point_direction;
       vector_proj_point = vector_match_point + ds * vector_match_point_direction;
       proj_heading = match_point_heading + match_point_kappa * ds;
       proj_kappa = match_point_kappa;
       %计算结果输出
       proj_x_set(i) = vector_proj_point(1);
       proj_y_set(i) = vector_proj_point(2);
       proj_heading_set(i) = proj_heading;
       proj_kappa_set(i) = proj_kappa;
  
    end
    %匹配点的计算结果保存，供下一个周期使用
    pre_match_point_index_set = match_point_index_set;
    pre_frenet_path_x = frenet_path_x;
    pre_frenet_path_y = frenet_path_y;
    pre_frenet_path_heading = frenet_path_heading;
    pre_frenet_path_kappa = frenet_path_kappa;
end

== matlab function testemplanner_cs/Audi_A8_Sedan_1/decision&planning module/EM_planner1/calc path length and map between point and s ==
  data: trajectory_x input; path_s_end output; trajectory_y input; path_s output
function [path_s_end,path_s] = fcn(trajectory_x,trajectory_y)
% 该函数将计算以trajectory的s 与 x y 的对应关系，可以看作是trajectory index2s
n = length(trajectory_x);
path_s = zeros(n,1);
sum = 0;
for i = 2:length(trajectory_x)
    if isnan(trajectory_x(i))
        break;
    end
    sum = sum + sqrt((trajectory_x(i) - trajectory_x(i-1))^2 + (trajectory_y(i) - trajectory_y(i-1))^2);
    path_s(i) = sum;
end
% 计算出trajectory的长度
if i == n
    path_s_end = path_s(end);
else
    % 因为循环的退出条件为isnan(trajectory_x(i)) 所以 i 所对应的数为 nan 
    path_s_end = path_s(i - 1);
end

== matlab function testemplanner_cs/Audi_A8_Sedan_1/decision&planning module/EM_planner1/calc plan start and stitch trajectory ==
  data: host_x input; plan_start_x output; host_y input; host_heading_xy input; host_vx input; host_vy input; host_ax input; host_ay input; pre_trajectory_x input; pre_trajectory_y input; pre_trajectory_heading input; pre_trajectory_kappa input; pre_trajectory_velocity input; pre_trajectory_accelerate input; pre_trajectory_time input; current_time input; plan_start_y output; plan_start_heading output; plan_start_kappa output; plan_start_vx output; plan_start_vy output; plan_start_ax output; plan_start_ay output; plan_start_time output; stitch_x output; stitch_y output; stitch_heading output; stitch_kappa output; stitch_velocity output; stitch_accelerate output; stitch_time output
function [plan_start_x,plan_start_y,plan_start_heading,plan_start_kappa,plan_start_vx,plan_start_vy,plan_start_ax,plan_start_ay,plan_start_time,stitch_x,stitch_y,...
    stitch_heading,stitch_kappa,stitch_velocity,stitch_accelerate,stitch_time] = fcn(host_x,host_y,host_heading_xy,host_vx,host_vy,host_ax,host_ay,pre_trajectory_x,pre_trajectory_y,...
    pre_trajectory_heading,pre_trajectory_kappa,pre_trajectory_velocity,pre_trajectory_accelerate,pre_trajectory_time,current_time)

%%作用：求得当前周期的规划起点，有两种方式，①一种方式是车辆当前位置与上一周期规划路径点相差较大，此时需要通过车辆动力学外推得到，②另一种方式是相差不大，直径将原有路径延长得到
%%输入：上一个周期规划出的路径的坐标点，航向，速度，加速度。车辆当前的坐标点、航向，速度，加速度，当前时间。
%%输出；规划起点的坐标点，航向，速度，加速度；待拼接轨迹的坐标点，航向，速度，加速度以及时间。

% 初始化待拼接轨迹，此轨迹主要用来进行拼接，加速计算过程，待拼接轨迹为计算的规划起点在原有轨迹上的位置向前取20个点，因此初始化一个20个点的数组
stitch_x=zeros(20,1)*nan;
stitch_y=zeros(20,1)*nan;
stitch_heading=zeros(20,1)*nan;
stitch_kappa=zeros(20,1)*nan;
stitch_velocity=zeros(20,1)*nan;
stitch_accelerate=zeros(20,1)*nan;
%时间初始化为-1，代表没有要拼接的轨迹
stitch_time=ones(20,1)*(-1);

%根据是否为第一次运行进行区分，
persistent is_first_run

if isempty(is_first_run)
    %算法首次运行，本来需要外推，但因为是首次运行就以车辆当前的位置作为规划起点
    is_first_run=0;
    plan_start_x=host_x;
    plan_start_y=host_y;
    plan_start_heading=host_heading_xy;
    plan_start_kappa=0;
    plan_start_vx=0;
    plan_start_vy=0;
    plan_start_ax=0;
    plan_start_ay=0;
    %规划起点时间戳为当前时间+100ms
    plan_start_time=current_time+0.1;
else
    %算法不是首次运行，可以正常运行
    
    %比较车辆当前实际位置与车辆规划位置的差别
    
    x_current=host_x;
    y_current=host_y;
    heading_current=host_heading_xy;
    kappa_current=0;%默认起点曲率为0
    %要转换为世界坐标系
    vx_current=host_vx*cos(heading_current)-host_vy*sin(heading_current);
    vy_current=host_vx*sin(heading_current)+host_vy*cos(heading_current);
    ax_current=host_ax*cos(heading_current)-host_ay*sin(heading_current);
    ay_current=host_ax*sin(heading_current)+host_ay*cos(heading_current);
    %接着遍历数组，求解根据规划，车辆当前应道在的位置
    for i=1:length(pre_trajectory_time)
        if(pre_trajectory_time(i)<=current_time)&&(pre_trajectory_time(i+1)>current_time)
           break; 
        else
        end
    end
    x_desire=pre_trajectory_x(i);
    y_desire=pre_trajectory_x(i);
    heading_desire=pre_trajectory_heading(i);
%     vx_desire=pre_trajectory_velocity*cos(pre_trajectory_heading(i));
%     vy_desire=pre_trajectory_velocity*sin(pre_trajectory_heading(i));
%     ax_desire=pre_trajectory_accelerate*cos(pre_trajectory_heading(i));
%     ay_desire=pre_trajectory_accelerate*sin(pre_trajectory_heading(i));
    
   %得到两个位置的误差
   %通过向量法计算误差
   %切向向量
   tor = [cos(heading_desire);sin(heading_desire)];
   %法向向量
   nor = [-sin(heading_desire);cos(heading_desire)];
   %两点向量
   error = [host_x;host_y]-[x_desire;y_desire];
   %纵向误差
   long_error = abs(error'*tor);
   %横向误差
   lat_error = abs(error'*nor);
   
   if (long_error>2.5)||(lat_error>0.5)   %控制误差过大，使用车辆动力学外推
        dt=0.1;
        plan_start_x=x_current+vx_current*dt+0.5*ax_current*dt*dt;
        plan_start_y=y_current+vy_current*dt+0.5*ay_current*dt*dt;
        plan_start_kappa=kappa_current;
        plan_start_vx=vx_current+ax_current*dt;
        plan_start_vy=vy_current+ay_current*dt;
        plan_start_ax=ax_current;
        plan_start_ay=ax_current;
        plan_start_heading=atan2(plan_start_vy,plan_start_vx);
    %规划起点时间戳为当前时间+100ms
        plan_start_time=current_time+0.1;
   else     %控制误差不大，则利用上一个周期规划路径找点
       for j=i:length(pre_trajectory_time)
            if (pre_trajectory_time(j)<=current_time+0.1)&&(pre_trajectory_time(j+1)>current_time+0.1)
                break;
            end
       end
        plan_start_x=pre_trajectory_x(j);
        plan_start_y=pre_trajectory_y(j);
        plan_start_heading=pre_trajectory_heading(j);
        plan_start_kappa=pre_trajectory_kappa(j);
        plan_start_vx=pre_trajectory_velocity(j)*cos(pre_trajectory_heading(j));
        plan_start_vy=pre_trajectory_velocity(j)*sin(pre_trajectory_heading(j));
        % 注意，由于是做圆周运动，所以加速度要先按照切向和法相进行分解
         %切向向量
         tor = [cos(heading_desire);sin(heading_desire)];
         %法向向量
         nor = [-sin(heading_desire);cos(heading_desire)];
        tor_a=pre_trajectory_accelerate(j)*tor;        %切向加速度
        nor_a=pre_trajectory_velocity(j)*pre_trajectory_kappa(j)*nor; %法向加速度=v^2/r
        %分别将切向加速度和法向加速度的x，y分量相加就是ax和ay
        plan_start_ax=tor_a(1)+nor_a(1);
        plan_start_ay=tor_a(2)+nor_a(2);
    %规划起点时间戳为当前时间+100ms
        plan_start_time=pre_trajectory_time(j); 
         %下面开始进行轨迹拼接
         %当前节点是j，如果j大于20，则往前拼接20个点，如果j<20，则能拼几个点就拼几个点。从stitch最后一个点开始拼，没有拼上的点time为-1
%          if j>=21
%              for k=j-1:-1:j-20
%                  stitch_time(k)=pre_trajectory_time(k);
%                  stitch_x(k)=pre_trajectory_x(k);
%                  stitch_y(k)=pre_trajectory_y(k);
%                  stitch_heading(k)=pre_trajectory_heading(k);
%                  stitch_kappa(k)=pre_trajectory_kappa(k);
%                  stitch_velocity(k) = pre_trajectory_velocity(k);
%                  stitch_accelerate (k)= pre_trajectory_accelerate (k);
%              end
%          else
%              for k=1:j-1
%                  stitch_time(20+1-k)=pre_trajectory_time(j-k);
%                  stitch_x(20+1-k)=pre_trajectory_x(j-k);
%                  stitch_y(20+1-k)=pre_trajectory_y(j-k);
%                  stitch_heading(20+1-k)=pre_trajectory_heading(j-k);
%                  stitch_kappa(20+1-k)=pre_trajectory_kappa(j-k);
%                  stitch_velocity(20+1-k) = pre_trajectory_velocity(j-k);
%                  stitch_accelerate(20+1-k) = pre_trajectory_accelerate(j-k);
%              end
%          end
 j = j - 1;
        if j >= 20
            stitch_x = pre_trajectory_x(j - 19:j);
            stitch_y = pre_trajectory_y(j - 19:j);
            stitch_heading = pre_trajectory_heading(j - 19:j);
            stitch_kappa = pre_trajectory_kappa(j - 19:j);
            stitch_velocity = pre_trajectory_velocity(j - 19:j);
            stitch_accelerate = pre_trajectory_accelerate(j - 19:j);
            stitch_time = pre_trajectory_time(j - 19:j);
        else
            stitch_x(20 - j + 1:20) = pre_trajectory_x(1:j);
            stitch_y(20 - j + 1:20) = pre_trajectory_y(1:j);
            stitch_heading(20 - j + 1:20) = pre_trajectory_heading(1:j);
            stitch_kappa(20 - j + 1:20) = pre_trajectory_kappa(1:j);
            stitch_accelerate(20 - j + 1:20) = pre_trajectory_velocity(1:j);
            stitch_accelerate(20 - j + 1:20) = pre_trajectory_accelerate(1:j);
            stitch_time(20 - j + 1:20) = pre_trajectory_time(1:j);           
        end   
   end
   
   
   
end
